simulink model "es2V1"  (R2024a)
settings: Solver=VariableStepAuto  StartTime=0.0  StopTime=30  RelTol=1e-3
libraries: vrlib x3
settings Model: Creator=andre  LastModifiedBy=andre

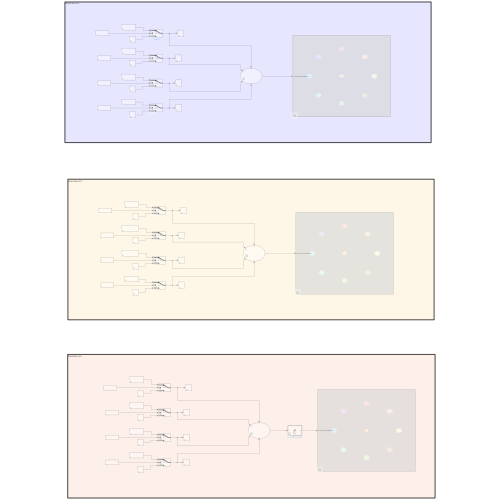
[thumbnail: Simulink's stored preview of the top-level diagram]
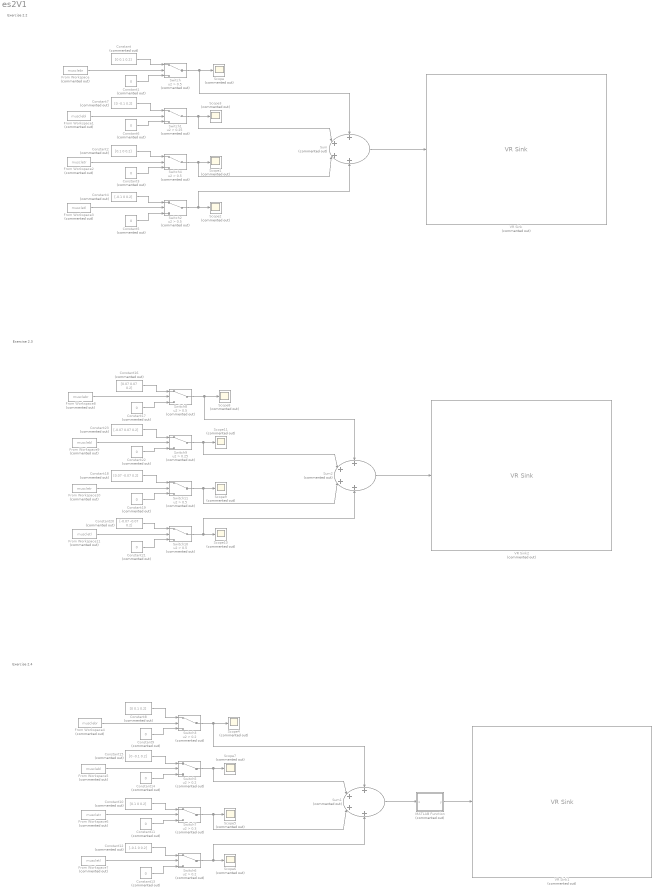
== system es2V1 ==
  note: Exercise 2.4
  note: Exercise 2.2
  note: Exercise 2.3
  Constant : Constant  Commented=on  Value=[0 0.1 0.2]
  Constant{1,3,5..6,9,11,13..14,17,19,21..22} (12 alike) : Constant  Commented=on  Value=0
  Constant10 : Constant  Commented=on  Value=[0.1 0 0.2]
  Constant12 : Constant  Commented=on  Value=[-0.1 0 0.2]
  Constant15 : Constant  Commented=on  Value=[0 -0.1 0.2]
  Constant16 : Constant  Commented=on  Value=[0.07 0.07 0.2]
  Constant18 : Constant  Commented=on  Value=[0.07 -0.07 0.2]
  Constant2 : Constant  Commented=on  Value=[0.1 0 0.2]
  Constant20 : Constant  Commented=on  Value=[-0.07 -0.07 0.2]
  Constant23 : Constant  Commented=on  Value=[-0.07 0.07 0.2]
  Constant4 : Constant  Commented=on  Value=[-0.1 0 0.2]
  Constant7 : Constant  Commented=on  Value=[0 -0.1 0.2]
  Constant8 : Constant  Commented=on  Value=[0 0.1 0.2]
  From Workspace : FromWorkspace  Commented=on  VariableName=musclebr  SampleTime=0.05
  From Workspace1 : FromWorkspace  Commented=on  VariableName=musclebl  SampleTime=0.05
  From Workspace10 : FromWorkspace  Commented=on  VariableName=muscletr  SampleTime=0.05
  From Workspace11 : FromWorkspace  Commented=on  VariableName=muscletl  SampleTime=0.05
  From Workspace2 : FromWorkspace  Commented=on  VariableName=muscletr  SampleTime=0.05
  From Workspace3 : FromWorkspace  Commented=on  VariableName=muscletl  SampleTime=0.05
  From Workspace4 : FromWorkspace  Commented=on  VariableName=musclebr  SampleTime=0.05
  From Workspace5 : FromWorkspace  Commented=on  VariableName=musclebl  SampleTime=0.05
  From Workspace6 : FromWorkspace  Commented=on  VariableName=muscletr  SampleTime=0.05
  From Workspace7 : FromWorkspace  Commented=on  VariableName=muscletl  SampleTime=0.05
  From Workspace8 : FromWorkspace  Commented=on  VariableName=musclebr  SampleTime=0.05
  From Workspace9 : FromWorkspace  Commented=on  VariableName=musclebl  SampleTime=0.05
  MATLAB Function : MATLAB Function  Commented=on  TreatAsAtomicUnit=on
  Scope{,1..11} (12 alike) : Scope  Commented=on
  Sum : Sum  Commented=on  Inputs=++++
  Sum1 : Sum  Commented=on  Inputs=++++
  Sum2 : Sum  Commented=on  Inputs=++++
  Switch{,2,4,8,10..11} (6 alike) : Switch  Commented=on  Criteria=u2 > Threshold  Threshold=0.5  SaturateOnIntegerOverflow=off  InputSameDT=off
  Switch1 : Switch  Commented=on  Criteria=u2 > Threshold  Threshold=0.25  SaturateOnIntegerOverflow=off  InputSameDT=off
  Switch3 : Switch  Commented=on  Criteria=u2 > Threshold  Threshold=0.2  SaturateOnIntegerOverflow=off  InputSameDT=off
  Switch5 : Switch  Commented=on  Criteria=u2 > Threshold  Threshold=0.2  SaturateOnIntegerOverflow=off  InputSameDT=off
  Switch6 : Switch  Commented=on  Criteria=u2 > Threshold  Threshold=0.2  SaturateOnIntegerOverflow=off  InputSameDT=off
  Switch7 : Switch  Commented=on  Criteria=u2 > Threshold  Threshold=0.3  SaturateOnIntegerOverflow=off  InputSameDT=off
  Switch9 : Switch  Commented=on  Criteria=u2 > Threshold  Threshold=0.25  SaturateOnIntegerOverflow=off  InputSameDT=off
  VR Sink : vrlib/VR Sink  Commented=on  InstantiateOnLoad=on  SampleTime=0.05  ViewEnable=on  RemoteChange=off  RemoteView=off  FieldsWritten=cursor.translation.3.1.1.double  WorldFileName=8_palline_color.wrl  AutoView=off  VideoDimensions=[]  AllowVariableSize=off
  VR Sink1 : vrlib/VR Sink  Commented=on  InstantiateOnLoad=on  SampleTime=0.005  ViewEnable=on  RemoteChange=off  RemoteView=off  FieldsWritten=cursor.translation.3.1.1.double  WorldFileName=8_palline_color.wrl  AutoView=off  VideoDimensions=[]  AllowVariableSize=off
  VR Sink2 : vrlib/VR Sink  Commented=on  InstantiateOnLoad=on  SampleTime=0.05  ViewEnable=on  RemoteChange=off  RemoteView=off  FieldsWritten=cursor.translation.3.1.1.double  WorldFileName=8_palline_color.wrl  AutoView=off  VideoDimensions=[]  AllowVariableSize=off
  wires:
  From Workspace1/1 -> Switch1/2
  From Workspace/1 -> Switch/2
  Switch/1 -> Sum/1, Scope/1
  Constant/1 -> Switch/1
  Constant1/1 -> Switch/3
  From Workspace2/1 -> Switch4/2
  Constant3/1 -> Switch4/3
  Switch4/1 -> Sum/3, Scope1/1
  Constant2/1 -> Switch4/1
  From Workspace3/1 -> Switch2/2
  Constant5/1 -> Switch2/3
  Switch2/1 -> Sum/4, Scope2/1
  Constant4/1 -> Switch2/1
  Constant6/1 -> Switch1/3
  Constant7/1 -> Switch1/1
  Switch1/1 -> Sum/2, Scope3/1
  Sum/1 -> VR Sink/1
  From Workspace7/1 -> Switch6/2
  Switch7/1 -> Sum1/3, Scope5/1
  Constant15/1 -> Switch5/1
  Constant10/1 -> Switch7/1
  Switch6/1 -> Sum1/4, Scope6/1
  Constant11/1 -> Switch7/3
  Constant8/1 -> Switch3/1
  Constant12/1 -> Switch6/1
  Constant14/1 -> Switch5/3
  Switch5/1 -> Sum1/2, Scope7/1
  Switch3/1 -> Sum1/1, Scope4/1
  From Workspace6/1 -> Switch7/2
  From Workspace4/1 -> Switch3/2
  Constant13/1 -> Switch6/3
  Constant9/1 -> Switch3/3
  From Workspace5/1 -> Switch5/2
  Sum1/1 -> MATLAB Function/1(x)
  MATLAB Function/1(y) -> VR Sink1/1
  Switch9/1 -> Sum2/2, Scope11/1
  Sum2/1 -> VR Sink2/1
  Switch11/1 -> Sum2/3, Scope9/1
  Constant18/1 -> Switch11/1
  Constant20/1 -> Switch10/1
  Constant22/1 -> Switch9/3
  Switch10/1 -> Sum2/4, Scope10/1
  From Workspace10/1 -> Switch11/2
  Constant19/1 -> Switch11/3
  Constant16/1 -> Switch8/1
  Constant21/1 -> Switch10/3
  Constant23/1 -> Switch9/1
  From Workspace9/1 -> Switch9/2
  From Workspace8/1 -> Switch8/2
  Constant17/1 -> Switch8/3
  From Workspace11/1 -> Switch10/2
  Switch8/1 -> Sum2/1, Scope8/1

== matlab function es2V1/MATLAB Function ==
  data: x input; y output
function y = fcn(x)
      
    if x(1)^2 + x(2)^2 <= 0.1^2
        y = [x(1), x(2), 0.2]; % Mantieni dimensioni fisse
    elseif x(1) > 0.01 && x(2) > 0.01 % caso primo quadrante
        y = [0.07, 0.07, 0.2];
    elseif x(1) < 0.01 && x(2) > 0.01 % caso secondo quadrante
        y = [-0.07, 0.07, 0.2];
    elseif x(1) < 0.01 && x(2) < 0.01 % caso terzo quadrante
        y = [-0.07, -0.07, 0.2];
    elseif x(1) > 0.01 && x(2) < 0.01 % caso quarto quadrante
        y = [0.07, -0.07, 0.2];
    else
        y = [x(1), x(2), 0.2]; % Mantieni dimensioni fisse
    end
end
